simulink model "model_problem6"  (R2020a)
settings: Solver=VariableStepAuto  StartTime=0.0  StopTime=10.0  RelTol=1e-3
settings Model: Creator=Prateek  LastModifiedBy=Prateek

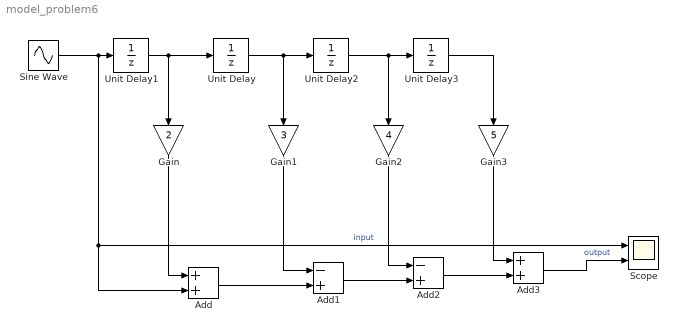
== system model_problem6 ==
  Add : Sum
  Add1 : Sum  Inputs=-+
  Add2 : Sum  Inputs=-+
  Add3 : Sum
  Gain : Gain  Gain=2
  Gain1 : Gain  Gain=3
  Gain2 : Gain  Gain=4
  Gain3 : Gain  Gain=5
  Scope : Scope  NumInputPorts=2
  Sine Wave : Sin  SampleTime=0
  Unit Delay{,1..3} (4 alike) : UnitDelay  SampleTime=-1  HasFrameUpgradeWarning=on
  wires:
  Sine Wave/1 -> Scope/1, Add/2, Unit Delay1/1  "input"
  Unit Delay1/1 -> Unit Delay/1, Gain/1
  Gain/1 -> Add/1
  Unit Delay/1 -> Gain1/1, Unit Delay2/1
  Unit Delay2/1 -> Gain2/1, Unit Delay3/1
  Add/1 -> Add1/2
  Gain1/1 -> Add1/1
  Add1/1 -> Add2/2
  Gain2/1 -> Add2/1
  Unit Delay3/1 -> Gain3/1
  Add2/1 -> Add3/2
  Gain3/1 -> Add3/1
  Add3/1 -> Scope/2  "output"
